simulink model "pid_discreto"  (R2025b)
settings: Solver=VariableStepAuto  StartTime=0.0  StopTime=10  RelTol=1e-3
undefined symbols (not defined in the file): DiscIntNeverNeededParam
libraries: simulink x6
settings Model: Creator=rel  LastModifiedBy=rel

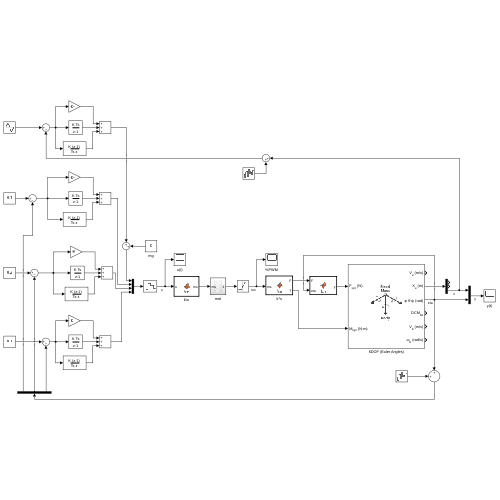
[thumbnail: Simulink's stored preview of the top-level diagram]
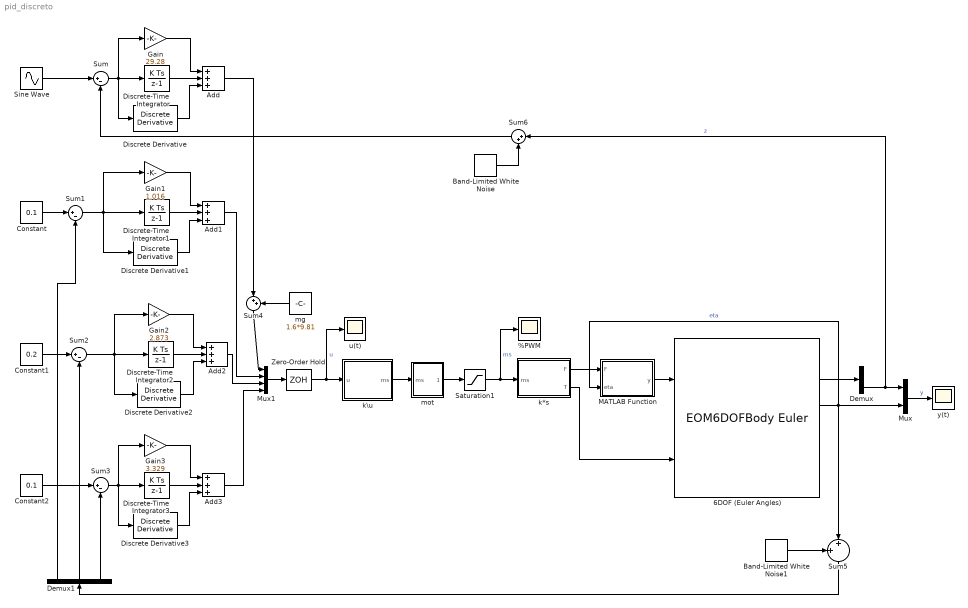
== system pid_discreto ==
  %PWM : Scope
      settings: ActiveDisplayYMinimum=-1  ActiveDisplayYMaximum=1  DataLoggingVariableName=ScopeData4
  6DOF (Euler Angles) : EOM6DOFBodyEuler  mass_0=1.6  inertia=diag([0.021915027 0.022124548 0.042349865])
  Add{,1..3} (4 alike) : Sum  Inputs=+++
  Band-Limited White Noise : simulink/Sources/Band-Limited White Noise  Cov=[0.0001]  Ts=0.1  seed=[23341]
  Band-Limited White Noise1 : simulink/Sources/Band-Limited White Noise  Cov=[0.0001]  Ts=0.1  seed=[23341]
  Constant : Constant  Value=0.1
  Constant1 : Constant  Value=0.2
  Constant2 : Constant  Value=0.1
  Demux : Demux  Outputs=3
  Demux1 : Demux  Outputs=3
  Discrete Derivative : simulink/Discrete/Discrete Derivative  gainval=38.21  ICPrevScaledInput=0.0  OutMin=[]  OutMax=[]  OutDataType=fixdt(1, 16)  OutScaling=2^-10  DoSatur=off
  Discrete Derivative1 : simulink/Discrete/Discrete Derivative  gainval=0.2  ICPrevScaledInput=0.0  OutMin=[]  OutMax=[]  OutDataType=fixdt(1, 16)  OutScaling=2^-10  DoSatur=off
  Discrete Derivative2 : simulink/Discrete/Discrete Derivative  gainval=0.6391  ICPrevScaledInput=0.0  OutMin=[]  OutMax=[]  OutDataType=fixdt(1, 16)  OutScaling=2^-10  DoSatur=off
  Discrete Derivative3 : simulink/Discrete/Discrete Derivative  gainval=2.288  ICPrevScaledInput=0.0  OutMin=[]  OutMax=[]  OutDataType=fixdt(1, 16)  OutScaling=2^-10  DoSatur=off
  Discrete-Time Integrator : DiscreteIntegrator  gainval=0.8  SampleTime=1/510  ICPrevOutput=DiscIntNeverNeededParam  ICPrevScaledInput=DiscIntNeverNeededParam
  Discrete-Time Integrator1 : DiscreteIntegrator  gainval=0.08  SampleTime=1/510  ICPrevOutput=DiscIntNeverNeededParam  ICPrevScaledInput=DiscIntNeverNeededParam
  Discrete-Time Integrator2 : DiscreteIntegrator  gainval=1.173  SampleTime=1/510  ICPrevOutput=DiscIntNeverNeededParam  ICPrevScaledInput=DiscIntNeverNeededParam
  Discrete-Time Integrator3 : DiscreteIntegrator  gainval=1.211  SampleTime=1/510  ICPrevOutput=DiscIntNeverNeededParam  ICPrevScaledInput=DiscIntNeverNeededParam
  Gain : Gain  Gain=29.28
  Gain1 : Gain  Gain=1.016
  Gain2 : Gain  Gain=2.873
  Gain3 : Gain  Gain=3.329
  MATLAB Function : MATLAB Function  TreatAsAtomicUnit=on
  Mux : Mux  Inputs=2
  Mux1 : Mux
  Saturation1 : Saturate  UpperLimit=1  LowerLimit=0
  Sine Wave : Sin  Amplitude=0.5  Bias=1  Frequency=2  SampleTime=0
  Sum{,1..3} (4 alike) : Sum  Inputs=|+-
  Sum4 : Sum  Inputs=|++
  Sum5 : Sum  Inputs=+|+||
  Sum6 : Sum  Inputs=|++
  Zero-Order Hold : ZeroOrderHold  SampleTime=1/510
  k*s : MATLAB Function  TreatAsAtomicUnit=on
  k\u : MATLAB Function  TreatAsAtomicUnit=on
  mg : Constant  Value=1.6*9.81
  mot : Subsystem
  u(t) : Scope
      settings: ActiveDisplayYMinimum=-193.56588912020933  ActiveDisplayYMaximum=176.54602226770902
  y(t) : Scope
      settings: ActiveDisplayYMinimum=-0.27700486996084006  ActiveDisplayYMaximum=1.6063695302954337
  wires:
  6DOF (Euler Angles)/2 -> Demux/1
  6DOF (Euler Angles)/3 -> Sum5/2, MATLAB Function/2(eta), Mux/2  "eta"
  mot/1(Out1) -> Saturation1/1
  k\u/1(ms) -> mot/1(ms)
  Saturation1/1 -> %PWM/1, k*s/1(ms)  "ms"
  k*s/2(T) -> 6DOF (Euler Angles)/2
  k*s/1(F) -> MATLAB Function/1(F)
  MATLAB Function/1(y) -> 6DOF (Euler Angles)/1
  Sum/1 -> Discrete-Time Integrator/1, Gain/1, Discrete Derivative/1
  Discrete Derivative/1 -> Add/3
  Gain/1 -> Add/1
  Mux1/1 -> Zero-Order Hold/1
  Zero-Order Hold/1 -> u(t)/1, k\u/1(u)  "u"
  Demux1/1 -> Sum1/2
  Demux1/2 -> Sum2/2
  Demux1/3 -> Sum3/2
  Demux/3 -> Sum6/1, Mux/1  "z"
  Mux/1 -> y(t)/1  "y"
  Sine Wave/1 -> Sum/1
  Constant1/1 -> Sum2/1
  Constant2/1 -> Sum3/1
  Constant/1 -> Sum1/1
  Add/1 -> Sum4/1
  Sum4/1 -> Mux1/1
  mg/1 -> Sum4/2
  Discrete-Time Integrator/1 -> Add/2
  Discrete Derivative1/1 -> Add1/3
  Discrete-Time Integrator1/1 -> Add1/2
  Gain1/1 -> Add1/1
  Sum1/1 -> Discrete Derivative1/1, Gain1/1, Discrete-Time Integrator1/1
  Discrete Derivative2/1 -> Add2/3
  Discrete-Time Integrator2/1 -> Add2/2
  Gain2/1 -> Add2/1
  Sum2/1 -> Gain2/1, Discrete Derivative2/1, Discrete-Time Integrator2/1
  Discrete Derivative3/1 -> Add3/3
  Discrete-Time Integrator3/1 -> Add3/2
  Gain3/1 -> Add3/1
  Sum3/1 -> Gain3/1, Discrete Derivative3/1, Discrete-Time Integrator3/1
  Add1/1 -> Mux1/2
  Add2/1 -> Mux1/3
  Add3/1 -> Mux1/4
  Band-Limited White Noise1/1 -> Sum5/1
  Sum5/1 -> Demux1/1
  Band-Limited White Noise/1 -> Sum6/2
  Sum6/1 -> Sum/2

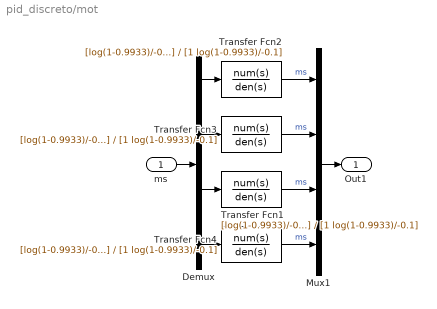
== system pid_discreto/mot ==
  ms : Inport
  Demux : Demux
  Mux1 : Mux
  Transfer Fcn{1..4} (4 alike) : TransferFcn  Numerator=[log(1-0.9933)/-0.1]  Denominator=[1 log(1-0.9933)/-0.1]
  Out1 : Outport
  wires:
  Transfer Fcn3/1 -> Mux1/2  "ms"
  Transfer Fcn1/1 -> Mux1/3  "ms"
  Demux/3 -> Transfer Fcn1/1
  Transfer Fcn4/1 -> Mux1/4  "ms"
  Demux/4 -> Transfer Fcn4/1
  Mux1/1 -> Out1/1
  Transfer Fcn2/1 -> Mux1/1  "ms"
  Demux/2 -> Transfer Fcn3/1
  Demux/1 -> Transfer Fcn2/1
  ms/1 -> Demux/1

== matlab function pid_discreto/k\u ==
  data: u input; ms output
function ms = fcn(u)
% L = 0.0080;
% kF = 0.1600*9.81;
% kM = 0.0086;
L = 0.268554;
kF = 0.7*9.81;
kM = 0.2;
A = [kF kF kF kF; -L*kF -L*kF L*kF L*kF; L*kF -L*kF -L*kF L*kF; -kM kM -kM kM];
ms = A\[u(1); u(2:end)];

== matlab function pid_discreto/MATLAB Function ==
  data: F input; y output; eta input
function y = fcn(F, eta)
phi = eta(1);
theta = eta(2);
psi = eta(3);
y = [0;0;-1.6*9.81] + [sin(theta)*cos(psi) + sin(phi)*cos(theta)*sin(psi); ...
                    sin(theta)*sin(psi) - sin(phi)*cos(theta)*cos(psi); ...
                    cos(phi)*cos(theta)]*F;

== matlab function pid_discreto/k*s ==
  data: ms input; F output; T output
function [F, T] = fcn(ms)
% L = 0.0080;
% kF = 0.1600*9.81;
% kM = 0.0086;
L = 0.268554;
kF = 0.7*9.81;
kM = 0.2;
A = [kF kF kF kF; -L*kF -L*kF L*kF L*kF; L*kF -L*kF -L*kF L*kF; -kM kM -kM kM];
y = A*ms;
F = y(1);
T = y(2:end);
